simulink model "test"  (Simulink 9.1)
settings: Solver=VariableStepAuto  StartTime=0.0  StopTime=inf  RelTol=1e-3
libraries: WBToolboxLibrary x4
settings Model: SuppressorTable=22 serialization::archive 11 0 6 0 0 0 1 0  Creator=yeshi  LastModifiedBy=yeshi
settings DataIOCC: SaveFormat=Dataset
settings OptimizationCC: LifeSpan=auto
settings DebuggingCC: UnderspecifiedInitializationDetection=Simplified  MergeDetectMultiDrivingBlocksExec=error  SFUnexpectedBacktrackingDiag=error  SFNoUnconditionalDefaultTransitionDiag=error  SFExecutionAtInitializationDiag=warning
settings HardwareCC: ProdBitPerPointer=64  ProdBitPerSizeT=64  ProdBitPerPtrDiffT=64  ProdLargestAtomicFloat=Float  ProdIntDivRoundTo=Zero  ProdEndianess=LittleEndian  ProdWordSize=64  ProdHWDeviceType=Intel->x86-64 (Windows64)
settings ModelReferenceCC: PropagateSignalLabelsOutOfModel=on
settings CodeAppCC: StateflowObjectComments=off
settings GRTTargetCC: TargetLangStandard=C99 (ISO)  CombineOutputUpdateFcns=on  GRTInterface=off
settings ConfigComp: CovMetricSettings=dwe  CovHtmlReporting=off  CovSaveCumulativeToWorkspaceVar=off  CovSaveSingleToWorkspaceVar=off  CovExternalEMLEnable=on

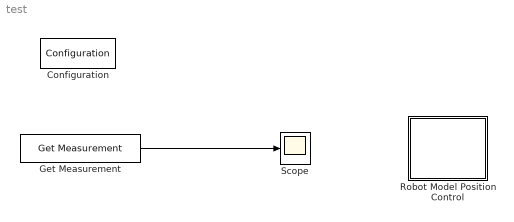
== system test ==
  Configuration : WBToolboxLibrary/Utilities/Configuration  ConfigSource=Mask  ConfigObject='HUMAN_WBTConfigRobot'  RobotName='icubSim'  UrdfFile='model.urdf'  ControlledJoints={'l_hip_pitch','l_hip_roll','l_hip_yaw','l_knee','l_ankle_pitch','l_ankle_roll','r_hip_pitch','r_hip_roll','r_hip_yaw','r_knee','r_ankle_pitch','r_ankle_roll'}  ControlBoardsNames={'left_leg','right_leg'}  LocalName='WBT'  GravityVector=[0,0,-9.81]
      settings: SourceProductName=Whole Body Toolbox
  Get Measurement : WBToolboxLibrary/wholeBodyStates/Get Measurement  measuredType=Joints Position
      settings: SourceProductName=Whole Body Toolbox
  Robot Model Position Control : Subsystem
  Scope : Scope
  wires:
  Get Measurement/1 -> Scope/1

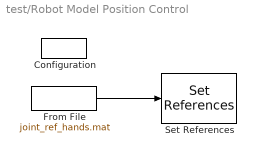
== system test/Robot Model Position Control ==
  Configuration : WBToolboxLibrary/Utilities/Configuration  ConfigSource=Mask  ConfigObject='HUMAN_WBTConfigRobot'  RobotName='icubSim'  UrdfFile='model.urdf'  ControlledJoints={'torso_pitch','torso_roll','torso_yaw','l_shoulder_pitch','l_shoulder_roll','l_shoulder_yaw','l_elbow','r_shoulder_pitch','r_shoulder_roll','r_shoulder_yaw','r_elbow'}  ControlBoardsNames={'torso','left_arm','right_arm'}  LocalName='WBT_HANDS'  GravityVector=[0,0,-9.81]
      settings: SourceProductName=Whole Body Toolbox
  From File : FromFile  FileName=joint_ref_hands.mat  SampleTime=0
  Set References : WBToolboxLibrary/wholeBodyActuators/Set References  controlType=Position  refSpeed=10*(pi/180)  refAcceleration=1000000*(pi/180)
      settings: SourceProductName=Whole Body Toolbox
  wires:
  From File/1 -> Set References/1
